simulink model "WECS2_WTeam6"  (R2023b)
settings: Solver=VariableStepAuto  StartTime=0.0  StopTime=6  RelTol=1e-3
undefined symbols (not defined in the file or in its folder): cP, D, fs, Fs_b, fsw, i_g, Ir_stator_b, Is_b, J, k_opt_hs, ki_id, ki_iq, ki_n, kp_id, kp_iq, kp_n, l_b, lambda, lambda_opt, Lm, Lr, Ls, Lsi, ns, p, Ps_b, rho_air, Rr, Rs, s_ini, sigma, theta_us_ini, Tm_b, Vbus, Vr_stator_b, Vs, Vs_b
libraries: slpidlib x3, spsThreePhaseVIMeasurementLib x2, spsAsynchronousMachineSIUnitsLib x1, spsabctoAlphaBetaZeroLib x1, spsabctodq0Lib x1, spsdq0toabcLib x1, spsDCVoltageSourceLib x1, spsGroundLib x1, spsPWMGenerator2LevelLib x1, sps_lib x1, spsThreePhaseProgrammableVoltageSourceLib x1, spsUniversalBridgeLib x1
settings Model: Creator=gauss  LastModifiedBy=smx
settings SolverCC: AlgebraicLoopSolver=TrustRegion
settings DebuggingCC: UnconnectedInputMsg=warning  UnconnectedOutputMsg=warning  UnconnectedLineMsg=warning
settings ModelReferenceCC: EnableRefExpFcnMdlSchedulingChecks=on
settings SFSimCC: CustomCodeUndefinedFunction=UseInterfaceOnly

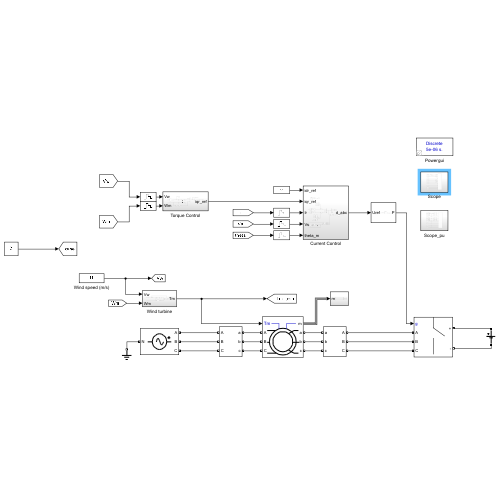
[thumbnail: Simulink's stored preview of the top-level diagram]
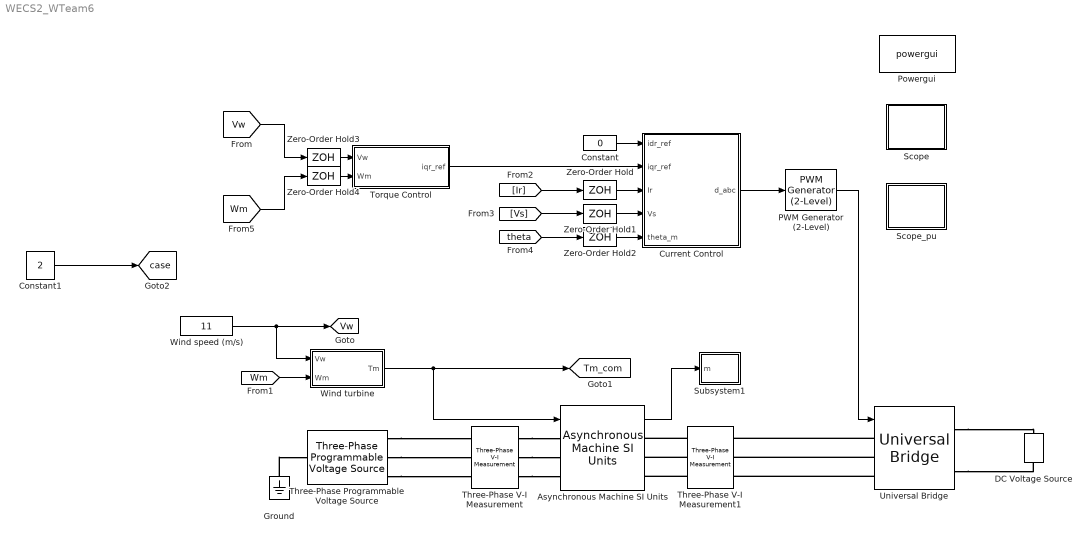
== system WECS2_WTeam6 ==
  Asynchronous Machine SI Units : spsAsynchronousMachineSIUnitsLib/Asynchronous Machine SI Units  RotorType=Wound  PresetModel=No  MechanicalLoad=Torque Tm  ShowDetailedParameters=on  ReferenceFrame=Rotor  Units=SI  MeasurementBus=off  NominalParameters=[Ps_b Vs fs]  VoltageRatio=1  Stator=[Rs Lsi]  Rotor=[Rr Lsi]  Cage1=[0.4155 0.002066]  Cage2=[0.4168 0.0003495]  Lm=Lm  Mechanical=[J D p]  PolePairs=2  InitialConditions=[s_ini 0 0 0 0 0 0 0 0 0 0 0 0 0]  SimulateSaturation=off  Saturation=[14.03593122, 27.81365428, 53.79336849, 72.68890987, 97.98006896, 148.6815601, 215.7428561, 302.9841135, 428.7778367 ; 230, 322, 414, 460, 506, 552, 598, 644, 690]  LoadFlowParameters=1492000  TsPowergui=0  TsBlock=-1  IterativeModel=Trapezoidal non iterative  IterativeDiscreteModel=Trapezoidal non iterative  Pmec=1.492e+006
  Constant : Constant  Value=0
  Constant1 : Constant  Value=2
  Current Control : Subsystem
  DC Voltage Source : spsDCVoltageSourceLib/DC Voltage Source  Amplitude=Vbus  Measurements=None
  Ground : spsGroundLib/Ground  LConnTagsString=a
  PWM Generator (2-Level) : spsPWMGenerator2LevelLib/PWM Generator (2-Level)  ModulatorType=Three-phase bridge (6 pulses)  ModulatorMode=Unsynchronized  Fc=fsw  Pc=90  nF=27  MinMax="[ -1  1 ]"  SamplingTechnique=Natural  ModulatingSignals=off  m=0.8  Freq=60  Phase=0  Ts=0  ShowCarrierOutport=off
  Powergui : sps_lib/powergui  Priority=1  SimulationMode=Discrete  SampleTime=5e-06  frequency=60  Iterations=50  frequencyindice=50  Pbase=100e6  ErrMax=1e-4  UnitsV=kV  UnitsW=MW  buscounter=0  FunctionMessages=off  echomessages=off  EnableUseOfTLC=off  CurrentSourceSwitches=off  DisableSnubberDevices=off  DisableRonSwitches=off  DisableVfSwitches=off  DisplayEquations=off  AutomaticDiscreteSolvers=off  SolverType=Tustin/Backward Euler (TBE)  Interpol=off  ExternalGateDelay=off  methode=off  Ts=100  x0status=blocks  SPID=on  SwTol=0  HookPort=off  NonlinearTolerance=1e-4  nMaxIteration=100  ContinueOnMaxIteration=off  RestoreLinks=warning  ResistiveCurrentMeasurement=off  Frange=[0:2:500]  Ylog=off  Xlog=on  ShowGrid=off  save=off  variable=ZData  structure=0  ZoomFFT=off  StartTime=0.0  cycles=1  DisplayStyle=1  fundamental=60  FreqAxis=off  MaxFrequency=1000  frequencyindicesteady=1  RmsSteady=1  display=off
  Scope : Subsystem
  Scope_pu : Subsystem
  Subsystem1 : Subsystem
  Three-Phase Programmable Voltage Source : spsThreePhaseProgrammableVoltageSourceLib/Three-Phase Programmable Voltage Source  PositiveSequence="[Vs  90-theta_us_ini fs]"  VariationEntity=None  VariationType=Table of time-amplitude pairs  VariationTypeAlt=Step  VariationStep=0.5  VariationRate=10  VariationMagnitude=0.3  VariationFrequency=2  VariationTiming=[1 2]  VariationPhaseA=off  Amplitudes=[1 0.8 1.2 1.0]  TimeValues=[0 0.1 0.15 0.2]  HarmonicGeneration=off  HarmonicA=[3 0.2 -25 0]  HarmonicB=[2 0.15 35 2]  Timing="[0.05  3]"  BusType=swing  Pref=0  Qref=0  Qmin=-inf  Qmax=inf
  Three-Phase V-I Measurement : spsThreePhaseVIMeasurementLib/Three-Phase V-I Measurement  VoltageMeasurement=phase-to-ground  SetLabelV=on  LabelV=Vs  Vpu=off  VpuLL=off  CurrentMeasurement=yes  SetLabelI=on  LabelI=Is  Ipu=off  Pbase=100e6  Vbase=500e3  OutputType=Complex  PhasorSimulation=off  PSBequivalent=0
  Three-Phase V-I Measurement1 : spsThreePhaseVIMeasurementLib/Three-Phase V-I Measurement  VoltageMeasurement=no  SetLabelV=off  LabelV=Vabc  Vpu=off  VpuLL=off  CurrentMeasurement=yes  SetLabelI=on  LabelI=Ir  Ipu=off  Pbase=100e6  Vbase=500e3  OutputType=Complex  PhasorSimulation=off  PSBequivalent=0
  Torque Control : Subsystem
  Universal Bridge : spsUniversalBridgeLib/Universal Bridge  Arms=3  SnubberResistance=1e5  SnubberCapacitance=inf  Device=Ideal Switches  Ron=1e-3  Lon=0  ForwardVoltages="[  0  0  ]"  ForwardVoltage=0  GTOparameters=[ 10e-6 , 20e-6 ]  IGBTparameters=[ 1e-6 , 2e-6 ]  Measurements=None  Measurements_2=None  converterType=Rectifier
  Wind speed (m/s) : Constant  Value=11
  Wind turbine : Subsystem
  Zero-Order Hold{,1..4} (5 alike) : ZeroOrderHold  SampleTime=-1
  tag scope: Tm_com=global, Vw=global, case=global
  wires:
  [Wm] -> Wind turbine/2(Wm)
  Wind speed (m/s)/1 -> Wind turbine/1(Vw), [Vw]
  Wind turbine/1(Tm) -> [Tm_com], Asynchronous Machine SI Units/1
  Asynchronous Machine SI Units/1 -> Subsystem1/1(m)
  PWM Generator (2-Level)/1 -> Universal Bridge/1
  Current Control/1(d_abc) -> PWM Generator (2-Level)/1
  Constant/1 -> Current Control/1(idr_ref)
  Zero-Order Hold/1 -> Current Control/3(Ir)
  Zero-Order Hold1/1 -> Current Control/4(Vs)
  Zero-Order Hold2/1 -> Current Control/5(theta_m)
  [Ir] -> Zero-Order Hold/1
  [Vs] -> Zero-Order Hold1/1
  [theta] -> Zero-Order Hold2/1
  Torque Control/1(iqr_ref) -> Current Control/2(iqr_ref)
  Zero-Order Hold3/1 -> Torque Control/1(Vw)
  Zero-Order Hold4/1 -> Torque Control/2(Wm)
  [Vw] -> Zero-Order Hold3/1
  [Wm] -> Zero-Order Hold4/1
  Constant1/1 -> [case]
  connections:
  Three-Phase V-I Measurement/RConn3 -- Asynchronous Machine SI Units/LConn3
  Three-Phase V-I Measurement/RConn2 -- Asynchronous Machine SI Units/LConn2
  Three-Phase V-I Measurement/RConn1 -- Asynchronous Machine SI Units/LConn1
  Three-Phase V-I Measurement1/RConn1 -- Asynchronous Machine SI Units/RConn1
  Three-Phase V-I Measurement1/RConn2 -- Asynchronous Machine SI Units/RConn2
  Three-Phase V-I Measurement1/RConn3 -- Asynchronous Machine SI Units/RConn3
  Three-Phase Programmable Voltage Source/RConn1 -- Three-Phase V-I Measurement/LConn1
  Three-Phase Programmable Voltage Source/RConn2 -- Three-Phase V-I Measurement/LConn2
  Three-Phase Programmable Voltage Source/RConn3 -- Three-Phase V-I Measurement/LConn3
  Ground/LConn1 -- Three-Phase Programmable Voltage Source/LConn1
  Universal Bridge/LConn1 -- Three-Phase V-I Measurement1/LConn1
  Universal Bridge/LConn2 -- Three-Phase V-I Measurement1/LConn2
  Universal Bridge/LConn3 -- Three-Phase V-I Measurement1/LConn3
  Universal Bridge/RConn1 -- DC Voltage Source/RConn1
  Universal Bridge/RConn2 -- DC Voltage Source/LConn1

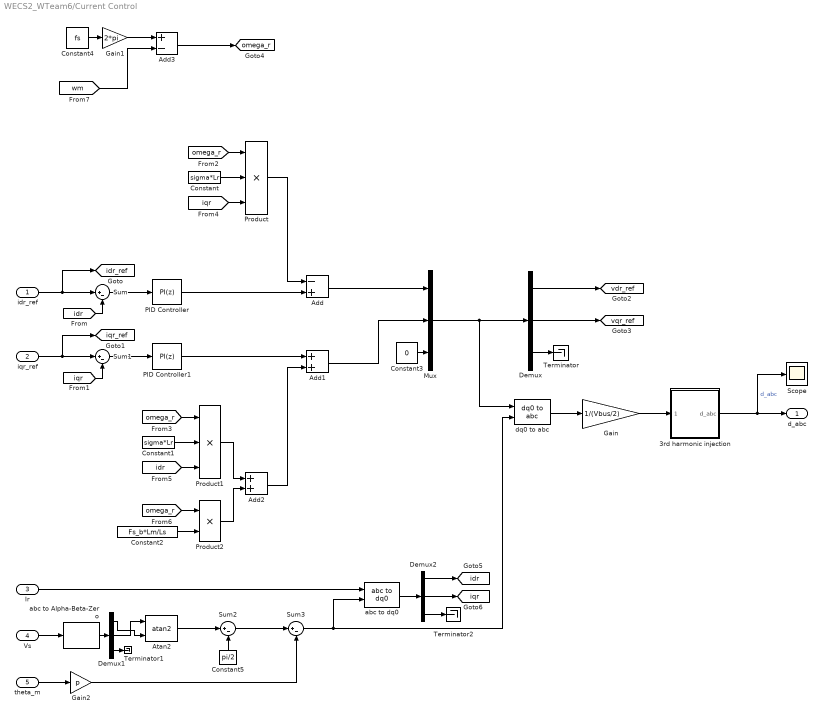
== system WECS2_WTeam6/Current Control ==
  idr_ref : Inport
  iqr_ref : Inport  Port=2
  Ir : Inport  Port=3
  Vs : Inport  Port=4
  theta_m : Inport  Port=5
  3rd harmonic injection : Subsystem
  Add : Sum  Inputs=-+
  Add1 : Sum
  Add2 : Sum
  Add3 : Sum  Inputs=+-
  Atan2 : Trigonometry  Operator=atan2
  Constant : Constant  Value=sigma*Lr
  Constant1 : Constant  Value=sigma*Lr
  Constant2 : Constant  Value=Fs_b*Lm/Ls
  Constant3 : Constant  Value=0
  Constant4 : Constant  Value=fs
  Constant5 : Constant  Value=pi/2
  Demux : Demux  Outputs=3
  Demux1 : Demux  Outputs=3
  Demux2 : Demux  Outputs=3
  Gain : Gain  Gain=1/(Vbus/2)
  Gain1 : Gain  Gain=2*pi
  Gain2 : Gain  Gain=p
  Mux : Mux  Inputs=3
  PID Controller : slpidlib/PID Controller  Controller=PI  Form=Parallel  TimeDomain=Discrete-time  UseExternalTs=off  SampleTime=1/fsw  IntegratorMethod=Forward Euler  FilterMethod=Forward Euler  ControllerParametersSource=internal  P=kp_id  I=ki_id  UseKiTs=off  D=0  N=100  UseFilter=on  TunerSelectOption=Transfer Function Based (PID Tuner App)  InitialConditionSource=internal  InitialConditionForIntegrator=0  InitialConditionForFilter=0  DifferentiatorICPrevScaledInput=0  ExternalReset=none  TrackingMode=off  Kt=1  LimitOutput=on  SatLimitsSource=internal  UpperSaturationLimit=Vbus/sqrt(3)  LowerSaturationLimit=-Vbus/sqrt(3)  LinearizeAsGain=on  AntiWindupMode=none  Kb=1  LimitIntegrator=off  UpperIntegratorSaturationLimit=inf  LowerIntegratorSaturationLimit=-inf  POutMin=[]  POutMax=[]  IOutMin=[]  IOutMax=[]  DOutMin=[]  DOutMax=[]  NOutMin=[]  NOutMax=[]  SumOutMin=[]  SumOutMax=[]  SaturationOutMin=[]  SaturationOutMax=[]  PParamMin=[]  PParamMax=[]  IParamMin=[]  IParamMax=[]  DParamMin=[]  DParamMax=[]  NParamMin=[]  NParamMax=[]  KbParamMin=[]  KbParamMax=[]  KtParamMin=[]  KtParamMax=[]  KbOutMin=[]  KbOutMax=[]  KtOutMin=[]  KtOutMax=[]  IntegratorOutMin=[]  IntegratorOutMax=[]  FilterOutMin=[]  FilterOutMax=[]  SumI1OutMin=[]  SumI1OutMax=[]  SumI2OutMin=[]  SumI2OutMax=[]  SumI3OutMin=[]  SumI3OutMax=[]  SumI4OutMin=[]  SumI4OutMax=[]  SumDOutMin=[]  SumDOutMax=[]  DifferentiatorOutMin=[]  DifferentiatorOutMax=[]  FilterDiffOutCoefMin=[]  FilterDiffOutCoefMax=[]  ReciprocalOutMin=[]  ReciprocalOutMax=[]  SumDenOutMin=[]  SumDenOutMax=[]  SumNumOutMin=[]  SumNumOutMax=[]  DivideOutMin=[]  DivideOutMax=[]  UdiffTsProdOutMin=[]  UdiffTsProdOutMax=[]  NTsProdOutMin=[]  NTsProdOutMax=[]  UintegralTsProdOutMin=[]  UintegralTsProdOutMax=[]  UngainTsProdOutMin=[]  UngainTsProdOutMax=[]  ClampingZeroOutDataTypeStr=Inherit: Inherit via back propagation  ClampingZeroOutMin=[]  ClampingZeroOutMax=[]  FilterDenConstantOutDataTypeStr=Inherit: Inherit via back propagation  FilterDenConstantOutMin=[]  FilterDenConstantOutMax=[]  PCopyOutDataTypeStr=Inherit: Inherit via back propagation  PCopyOutMin=[]  PCopyOutMax=[]  NCopyOutDataTypeStr=Inherit: Inherit via back propagation  NCopyOutMin=[]  NCopyOutMax=[]  IntegratorContinuousStateAttributes=''  IntegratorStateMustResolveToSignalObject=off  IntegratorRTWStateStorageClass=Auto  FilterContinuousStateAttributes=''  FilterStateMustResolveToSignalObject=off  FilterRTWStateStorageClass=Auto  ParallelPVariant=InternalParameters  IdealPVariant=Disabled  IVariant=InternalParameters  DVariant=Disabled  IntegratorVariant=Discrete  SatVariant=Enabled  AWVariant=Passthrough  PCopyVariant=Disabled  TRVariant=Disabled  FdbkBlocksVariant=Forward  IdealPFdbkVariant=Disabled  SatFdbkVariant=Disabled  DerivativeFilterVariant=Disabled  NVariant=Disabled  NCopyVariant=Disabled_SignalSpec  FilterICVariant=Disabled  IntegratorICVariant=InternalICs  ExternalResetVariant=Disabled  TRSumVariant=Passthrough  SumFdbkVariant=Disabled  SumVariant=Sum_PI  TsampFilterVariant=InternalTs  TsampNgainVariant=Passthrough  TsampIntegralVariant=Disabled_SignalSpec  ExternalSaturationOutDataTypeStr=Inherit: Same as second input
  PID Controller1 : slpidlib/PID Controller  Controller=PI  Form=Parallel  TimeDomain=Discrete-time  UseExternalTs=off  SampleTime=1/fsw  IntegratorMethod=Forward Euler  FilterMethod=Forward Euler  ControllerParametersSource=internal  P=kp_iq  I=ki_iq  UseKiTs=off  D=0  N=100  UseFilter=on  TunerSelectOption=Transfer Function Based (PID Tuner App)  InitialConditionSource=internal  InitialConditionForIntegrator=0  InitialConditionForFilter=0  DifferentiatorICPrevScaledInput=0  ExternalReset=none  TrackingMode=off  Kt=1  LimitOutput=on  SatLimitsSource=internal  UpperSaturationLimit=Vbus/sqrt(3)  LowerSaturationLimit=-Vbus/sqrt(3)  LinearizeAsGain=on  AntiWindupMode=none  Kb=1  LimitIntegrator=off  UpperIntegratorSaturationLimit=inf  LowerIntegratorSaturationLimit=-inf  POutMin=[]  POutMax=[]  IOutMin=[]  IOutMax=[]  DOutMin=[]  DOutMax=[]  NOutMin=[]  NOutMax=[]  SumOutMin=[]  SumOutMax=[]  SaturationOutMin=[]  SaturationOutMax=[]  PParamMin=[]  PParamMax=[]  IParamMin=[]  IParamMax=[]  DParamMin=[]  DParamMax=[]  NParamMin=[]  NParamMax=[]  KbParamMin=[]  KbParamMax=[]  KtParamMin=[]  KtParamMax=[]  KbOutMin=[]  KbOutMax=[]  KtOutMin=[]  KtOutMax=[]  IntegratorOutMin=[]  IntegratorOutMax=[]  FilterOutMin=[]  FilterOutMax=[]  SumI1OutMin=[]  SumI1OutMax=[]  SumI2OutMin=[]  SumI2OutMax=[]  SumI3OutMin=[]  SumI3OutMax=[]  SumI4OutMin=[]  SumI4OutMax=[]  SumDOutMin=[]  SumDOutMax=[]  DifferentiatorOutMin=[]  DifferentiatorOutMax=[]  FilterDiffOutCoefMin=[]  FilterDiffOutCoefMax=[]  ReciprocalOutMin=[]  ReciprocalOutMax=[]  SumDenOutMin=[]  SumDenOutMax=[]  SumNumOutMin=[]  SumNumOutMax=[]  DivideOutMin=[]  DivideOutMax=[]  UdiffTsProdOutMin=[]  UdiffTsProdOutMax=[]  NTsProdOutMin=[]  NTsProdOutMax=[]  UintegralTsProdOutMin=[]  UintegralTsProdOutMax=[]  UngainTsProdOutMin=[]  UngainTsProdOutMax=[]  ClampingZeroOutDataTypeStr=Inherit: Inherit via back propagation  ClampingZeroOutMin=[]  ClampingZeroOutMax=[]  FilterDenConstantOutDataTypeStr=Inherit: Inherit via back propagation  FilterDenConstantOutMin=[]  FilterDenConstantOutMax=[]  PCopyOutDataTypeStr=Inherit: Inherit via back propagation  PCopyOutMin=[]  PCopyOutMax=[]  NCopyOutDataTypeStr=Inherit: Inherit via back propagation  NCopyOutMin=[]  NCopyOutMax=[]  IntegratorContinuousStateAttributes=''  IntegratorStateMustResolveToSignalObject=off  IntegratorRTWStateStorageClass=Auto  FilterContinuousStateAttributes=''  FilterStateMustResolveToSignalObject=off  FilterRTWStateStorageClass=Auto  ParallelPVariant=InternalParameters  IdealPVariant=Disabled  IVariant=InternalParameters  DVariant=Disabled  IntegratorVariant=Discrete  SatVariant=Enabled  AWVariant=Passthrough  PCopyVariant=Disabled  TRVariant=Disabled  FdbkBlocksVariant=Forward  IdealPFdbkVariant=Disabled  SatFdbkVariant=Disabled  DerivativeFilterVariant=Disabled  NVariant=Disabled  NCopyVariant=Disabled_SignalSpec  FilterICVariant=Disabled  IntegratorICVariant=InternalICs  ExternalResetVariant=Disabled  TRSumVariant=Passthrough  SumFdbkVariant=Disabled  SumVariant=Sum_PI  TsampFilterVariant=InternalTs  TsampNgainVariant=Passthrough  TsampIntegralVariant=Disabled_SignalSpec  ExternalSaturationOutDataTypeStr=Inherit: Same as second input
  Product : Product  Inputs=3
  Product1 : Product  Inputs=3
  Product2 : Product
  Scope : Scope
  Sum{,1..3} (4 alike) : Sum  Inputs=|+-
  Terminator : Terminator
  Terminator1 : Terminator
  Terminator2 : Terminator
  abc to Alpha-Beta-Zero : spsabctoAlphaBetaZeroLib/abc to Alpha-Beta-Zero
  abc to dq0 : spsabctodq0Lib/abc to dq0  Alignment=Aligned with phase A axis
  dq0 to abc : spsdq0toabcLib/dq0 to abc  Alignment=Aligned with phase A axis
  d_abc : Outport
  tag scope: idr=global, idr_ref=global, iqr=global, iqr_ref=global, omega_r=global, vdr_ref=global, vqr_ref=global
  wires:
  idr_ref/1 -> [idr_ref], Sum/1
  [idr] -> Sum/2
  iqr_ref/1 -> [iqr_ref], Sum1/1
  [iqr] -> Sum1/2
  Sum/1 -> PID Controller/1
  Sum1/1 -> PID Controller1/1
  PID Controller/1 -> Add/2
  PID Controller1/1 -> Add1/1
  [iqr] -> Product/3
  Constant/1 -> Product/2
  [omega_r] -> Product/1
  Product/1 -> Add/1
  Constant1/1 -> Product1/2
  [idr] -> Product1/3
  [omega_r] -> Product1/1
  [omega_r] -> Product2/1
  Constant2/1 -> Product2/2
  Product1/1 -> Add2/1
  Product2/1 -> Add2/2
  Add2/1 -> Add1/2
  Add/1 -> Mux/1
  Add1/1 -> Mux/2
  Constant3/1 -> Mux/3
  Mux/1 -> dq0 to abc/1, Demux/1
  Demux/1 -> [vdr_ref]
  Demux/2 -> [vqr_ref]
  Demux/3 -> Terminator/1
  dq0 to abc/1 -> Gain/1
  Gain/1 -> 3rd harmonic injection/1(d_abc1)
  3rd harmonic injection/1(d_abc) -> Scope/1, d_abc/1  "d_abc"
  [wm] -> Add3/2
  Gain1/1 -> Add3/1
  Constant4/1 -> Gain1/1
  Add3/1 -> [omega_r]
  theta_m/1 -> Gain2/1
  Vs/1 -> abc to Alpha-Beta-Zero/1
  abc to Alpha-Beta-Zero/1 -> Demux1/1
  Demux1/3 -> Terminator1/1
  Demux1/2 -> Atan2/1
  Demux1/1 -> Atan2/2
  Atan2/1 -> Sum2/1
  Constant5/1 -> Sum2/2
  Sum2/1 -> Sum3/1
  Gain2/1 -> Sum3/2
  Ir/1 -> abc to dq0/1
  Sum3/1 -> dq0 to abc/2, abc to dq0/2
  abc to dq0/1 -> Demux2/1
  Demux2/3 -> Terminator2/1
  Demux2/2 -> [iqr]
  Demux2/1 -> [idr]

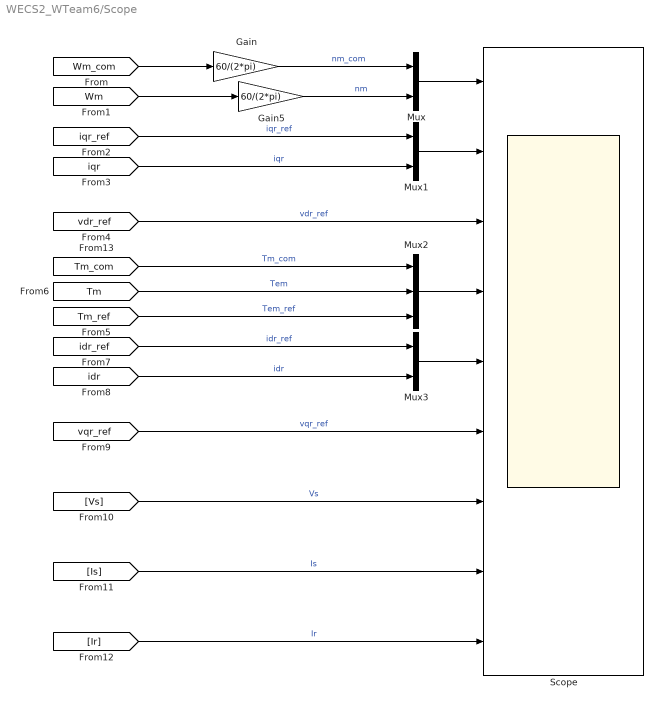
== system WECS2_WTeam6/Scope ==
  Gain : Gain  Gain=60/(2*pi)
  Gain5 : Gain  Gain=60/(2*pi)
  Mux : Mux  Inputs=2
  Mux1 : Mux  Inputs=2
  Mux2 : Mux  Inputs=3
  Mux3 : Mux  Inputs=2
  Scope : Scope  NumInputPorts=9
  wires:
  [Wm_com] -> Gain/1
  [Wm] -> Gain5/1
  Mux1/1 -> Scope/2
  [iqr_ref] -> Mux1/1  "iqr_ref"
  [iqr] -> Mux1/2  "iqr"
  [vdr_ref] -> Scope/3  "vdr_ref"
  [Tm] -> Mux2/2  "Tem"
  [idr] -> Mux3/2  "idr"
  Mux3/1 -> Scope/5
  [vqr_ref] -> Scope/6  "vqr_ref"
  [Vs] -> Scope/7  "Vs"
  [Is] -> Scope/8  "Is"
  [Ir] -> Scope/9  "Ir"
  Mux/1 -> Scope/1
  Mux2/1 -> Scope/4
  Gain/1 -> Mux/1  "nm_com"
  Gain5/1 -> Mux/2  "nm"
  [idr_ref] -> Mux3/1  "idr_ref"
  [Tm_ref] -> Mux2/3  "Tem_ref"
  [Tm_com] -> Mux2/1  "Tm_com"

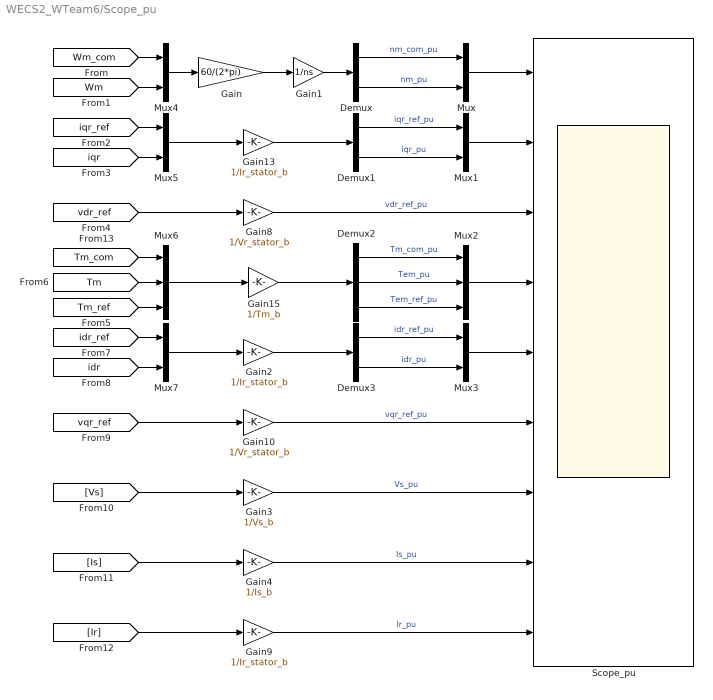
== system WECS2_WTeam6/Scope_pu ==
  Demux : Demux  Outputs=2
  Demux1 : Demux  Outputs=2
  Demux2 : Demux  Outputs=3
  Demux3 : Demux  Outputs=2
  Gain : Gain  Gain=60/(2*pi)
  Gain1 : Gain  Gain=1/ns
  Gain10 : Gain  Gain=1/Vr_stator_b
      settings: AttributesFormatString=%<Gain>
  Gain13 : Gain  Gain=1/Ir_stator_b
      settings: AttributesFormatString=%<Gain>
  Gain15 : Gain  Gain=1/Tm_b
      settings: AttributesFormatString=%<Gain>
  Gain2 : Gain  Gain=1/Ir_stator_b
      settings: AttributesFormatString=%<Gain>
  Gain3 : Gain  Gain=1/Vs_b
      settings: AttributesFormatString=%<Gain>
  Gain4 : Gain  Gain=1/Is_b
      settings: AttributesFormatString=%<Gain>
  Gain8 : Gain  Gain=1/Vr_stator_b
      settings: AttributesFormatString=%<Gain>
  Gain9 : Gain  Gain=1/Ir_stator_b
      settings: AttributesFormatString=%<Gain>
  Mux{,1,3..5,7} (6 alike) : Mux  Inputs=2
  Mux2 : Mux  Inputs=3
  Mux6 : Mux  Inputs=3
  "Scope_pu " : Scope  NumInputPorts=9
  wires:
  Mux1/1 -> "Scope_pu "/2
  [vdr_ref] -> Gain8/1
  Mux3/1 -> "Scope_pu "/5
  [vqr_ref] -> Gain10/1
  [Vs] -> Gain3/1
  [Is] -> Gain4/1
  [Ir] -> Gain9/1
  Mux/1 -> "Scope_pu "/1
  Mux2/1 -> "Scope_pu "/4
  Gain3/1 -> "Scope_pu "/7  "Vs_pu"
  Gain4/1 -> "Scope_pu "/8  "Is_pu"
  Demux/2 -> Mux/2  "nm_pu"
  Demux2/2 -> Mux2/2  "Tem_pu"
  Gain10/1 -> "Scope_pu "/6  "vqr_ref_pu"
  Gain8/1 -> "Scope_pu "/3  "vdr_ref_pu"
  Gain9/1 -> "Scope_pu "/9  "Ir_pu"
  Demux3/1 -> Mux3/1  "idr_ref_pu"
  Demux3/2 -> Mux3/2  "idr_pu"
  Demux1/1 -> Mux1/1  "iqr_ref_pu"
  Demux1/2 -> Mux1/2  "iqr_pu"
  Demux2/3 -> Mux2/3  "Tem_ref_pu"
  Demux2/1 -> Mux2/1  "Tm_com_pu"
  [Wm_com] -> Mux4/1
  [Wm] -> Mux4/2
  Mux4/1 -> Gain/1
  Gain/1 -> Gain1/1
  Demux/1 -> Mux/1  "nm_com_pu"
  Gain1/1 -> Demux/1
  Gain13/1 -> Demux1/1
  [iqr_ref] -> Mux5/1
  [iqr] -> Mux5/2
  Mux5/1 -> Gain13/1
  [Tm_ref] -> Mux6/3
  [Tm] -> Mux6/2
  [Tm_com] -> Mux6/1
  Mux6/1 -> Gain15/1
  Gain15/1 -> Demux2/1
  [idr] -> Mux7/2
  [idr_ref] -> Mux7/1
  Gain2/1 -> Demux3/1
  Mux7/1 -> Gain2/1

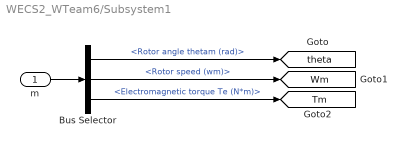
== system WECS2_WTeam6/Subsystem1 ==
  m : Inport
  Bus Selector : BusSelector  OutputSignals=Mechanical.Rotor angle thetam (rad),Mechanical.Rotor speed (wm),Mechanical.Electromagnetic torque Te (N*m)
  tag scope: Tm=global, Wm=global, theta=global
  wires:
  Bus Selector/2 -> [Wm]  "<Rotor speed (wm)>"
  Bus Selector/1 -> [theta]  "<Rotor angle thetam (rad)>"
  m/1 -> Bus Selector/1
  Bus Selector/3 -> [Tm]  "<Electromagnetic torque Te (N*m)>"

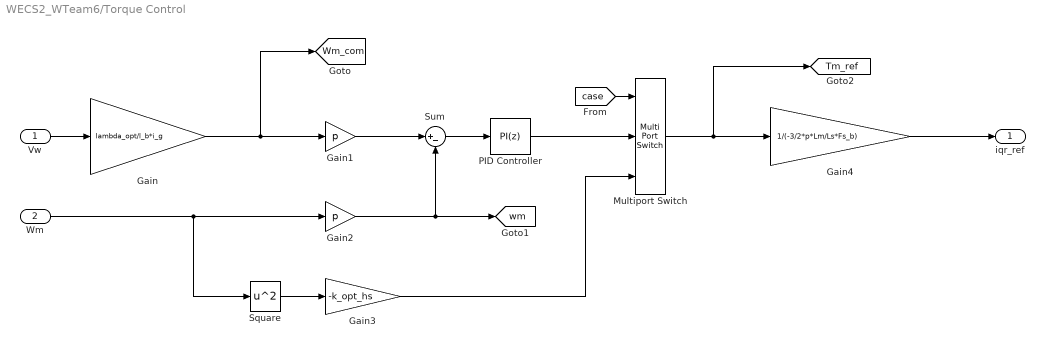
== system WECS2_WTeam6/Torque Control ==
  Vw : Inport
  Wm : Inport  Port=2
  Gain : Gain  Gain=lambda_opt/l_b*i_g
  Gain1 : Gain  Gain=p
  Gain2 : Gain  Gain=p
  Gain3 : Gain  Gain=-k_opt_hs
  Gain4 : Gain  Gain=1/(-3/2*p*Lm/Ls*Fs_b)
  Multiport Switch : MultiPortSwitch  Inputs=2  SaturateOnIntegerOverflow=off  InputSameDT=off
  PID Controller : slpidlib/PID Controller  Controller=PI  Form=Parallel  TimeDomain=Discrete-time  UseExternalTs=off  SampleTime=1/fsw  IntegratorMethod=Forward Euler  FilterMethod=Forward Euler  ControllerParametersSource=internal  P=kp_n  I=ki_n  UseKiTs=off  D=0  N=100  UseFilter=on  TunerSelectOption=Transfer Function Based (PID Tuner App)  InitialConditionSource=internal  InitialConditionForIntegrator=0  InitialConditionForFilter=0  DifferentiatorICPrevScaledInput=0  ExternalReset=none  TrackingMode=off  Kt=1  LimitOutput=on  SatLimitsSource=internal  UpperSaturationLimit=Tm_b  LowerSaturationLimit=-Tm_b  LinearizeAsGain=on  AntiWindupMode=none  Kb=1  LimitIntegrator=off  UpperIntegratorSaturationLimit=inf  LowerIntegratorSaturationLimit=-inf  POutMin=[]  POutMax=[]  IOutMin=[]  IOutMax=[]  DOutMin=[]  DOutMax=[]  NOutMin=[]  NOutMax=[]  SumOutMin=[]  SumOutMax=[]  SaturationOutMin=[]  SaturationOutMax=[]  PParamMin=[]  PParamMax=[]  IParamMin=[]  IParamMax=[]  DParamMin=[]  DParamMax=[]  NParamMin=[]  NParamMax=[]  KbParamMin=[]  KbParamMax=[]  KtParamMin=[]  KtParamMax=[]  KbOutMin=[]  KbOutMax=[]  KtOutMin=[]  KtOutMax=[]  IntegratorOutMin=[]  IntegratorOutMax=[]  FilterOutMin=[]  FilterOutMax=[]  SumI1OutMin=[]  SumI1OutMax=[]  SumI2OutMin=[]  SumI2OutMax=[]  SumI3OutMin=[]  SumI3OutMax=[]  SumI4OutMin=[]  SumI4OutMax=[]  SumDOutMin=[]  SumDOutMax=[]  DifferentiatorOutMin=[]  DifferentiatorOutMax=[]  FilterDiffOutCoefMin=[]  FilterDiffOutCoefMax=[]  ReciprocalOutMin=[]  ReciprocalOutMax=[]  SumDenOutMin=[]  SumDenOutMax=[]  SumNumOutMin=[]  SumNumOutMax=[]  DivideOutMin=[]  DivideOutMax=[]  UdiffTsProdOutMin=[]  UdiffTsProdOutMax=[]  NTsProdOutMin=[]  NTsProdOutMax=[]  UintegralTsProdOutMin=[]  UintegralTsProdOutMax=[]  UngainTsProdOutMin=[]  UngainTsProdOutMax=[]  ClampingZeroOutDataTypeStr=Inherit: Inherit via back propagation  ClampingZeroOutMin=[]  ClampingZeroOutMax=[]  FilterDenConstantOutDataTypeStr=Inherit: Inherit via back propagation  FilterDenConstantOutMin=[]  FilterDenConstantOutMax=[]  PCopyOutDataTypeStr=Inherit: Inherit via back propagation  PCopyOutMin=[]  PCopyOutMax=[]  NCopyOutDataTypeStr=Inherit: Inherit via back propagation  NCopyOutMin=[]  NCopyOutMax=[]  IntegratorContinuousStateAttributes=''  IntegratorStateMustResolveToSignalObject=off  IntegratorRTWStateStorageClass=Auto  FilterContinuousStateAttributes=''  FilterStateMustResolveToSignalObject=off  FilterRTWStateStorageClass=Auto  ParallelPVariant=InternalParameters  IdealPVariant=Disabled  IVariant=InternalParameters  DVariant=Disabled  IntegratorVariant=Discrete  SatVariant=Enabled  AWVariant=Passthrough  PCopyVariant=Disabled  TRVariant=Disabled  FdbkBlocksVariant=Forward  IdealPFdbkVariant=Disabled  SatFdbkVariant=Disabled  DerivativeFilterVariant=Disabled  NVariant=Disabled  NCopyVariant=Disabled_SignalSpec  FilterICVariant=Disabled  IntegratorICVariant=InternalICs  ExternalResetVariant=Disabled  TRSumVariant=Passthrough  SumFdbkVariant=Disabled  SumVariant=Sum_PI  TsampFilterVariant=InternalTs  TsampNgainVariant=Passthrough  TsampIntegralVariant=Disabled_SignalSpec  ExternalSaturationOutDataTypeStr=Inherit: Same as second input
  Square : Math  Operator=square
  Sum : Sum  Inputs=|+-
  iqr_ref : Outport
  tag scope: Tm_ref=global, Wm_com=global, wm=global
  wires:
  Vw/1 -> Gain/1
  Gain/1 -> [Wm_com], Gain1/1
  Gain1/1 -> Sum/1
  Sum/1 -> PID Controller/1
  Gain2/1 -> [wm], Sum/2
  Wm/1 -> Square/1, Gain2/1
  Square/1 -> Gain3/1
  PID Controller/1 -> Multiport Switch/2
  Gain3/1 -> Multiport Switch/3
  [case] -> Multiport Switch/1
  Multiport Switch/1 -> [Tm_ref], Gain4/1
  Gain4/1 -> iqr_ref/1

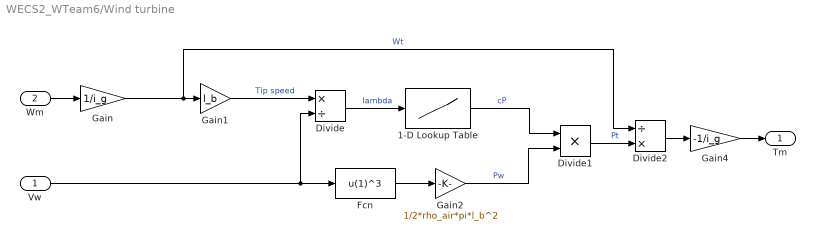
== system WECS2_WTeam6/Wind turbine ==
  Vw : Inport
  Wm : Inport  Port=2
  1-D Lookup Table : Lookup_n-D  NumberOfTableDimensions=1  BreakpointsForDimension1=lambda  BreakpointsForDimension1DataTypeStr=Inherit: Inherit from 'Breakpoint data'  Table=cP  TableDataTypeStr=Inherit: Inherit from 'Table data'  InternalRulePriority=Speed  RndMeth=Simplest
  Divide : Product  Inputs=*/
  Divide1 : Product  Inputs=**
  Divide2 : Product  Inputs=/*
  Fcn : Fcn  Expr=u(1)^3
  Gain : Gain  Gain=1/i_g
  Gain1 : Gain  Gain=l_b
  Gain2 : Gain  Gain=1/2*rho_air*pi*l_b^2
      settings: AttributesFormatString=%<Gain>
  Gain4 : Gain  Gain=-1/i_g
  Tm : Outport  VectorParamsAs1DForOutWhenUnconnected=off
  wires:
  Gain4/1 -> Tm/1
  Wm/1 -> Gain/1
  Gain/1 -> Divide2/1, Gain1/1  "Wt"
  Gain1/1 -> Divide/1  "Tip speed"
  Vw/1 -> Fcn/1, Divide/2
  Fcn/1 -> Gain2/1
  Gain2/1 -> Divide1/2  "Pw"
  Divide/1 -> 1-D Lookup Table/1  "lambda"
  1-D Lookup Table/1 -> Divide1/1  "cP"
  Divide1/1 -> Divide2/2  "Pt"
  Divide2/1 -> Gain4/1

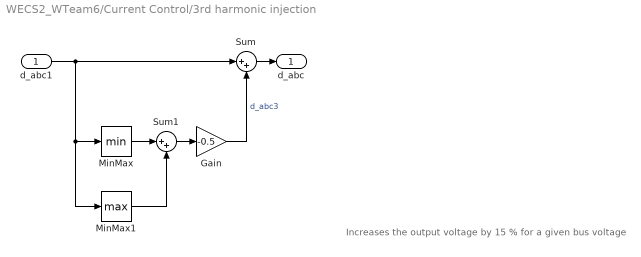
== system WECS2_WTeam6/Current Control/3rd harmonic injection ==
  note: Increases the output voltage by 15 % for a given bus voltage
  d_abc1 : Inport
  Gain : Gain  Gain=-0.5
  MinMax : MinMax
  MinMax1 : MinMax  Function=max
  Sum : Sum  Inputs=|++
  Sum1 : Sum  Inputs=|++
  d_abc : Outport  VectorParamsAs1DForOutWhenUnconnected=off
  wires:
  Sum/1 -> d_abc/1
  Gain/1 -> Sum/2  "d_abc3"
  d_abc1/1 -> Sum/1, MinMax1/1, MinMax/1
  MinMax/1 -> Sum1/1
  MinMax1/1 -> Sum1/2
  Sum1/1 -> Gain/1
